simulink model "coffe"  (R2015a)
settings: Solver=ode45  StartTime=0.0  StopTime=10.0  RelTol=1e-3
settings Model: Creator=lenovo  LastModifiedBy=lenovo

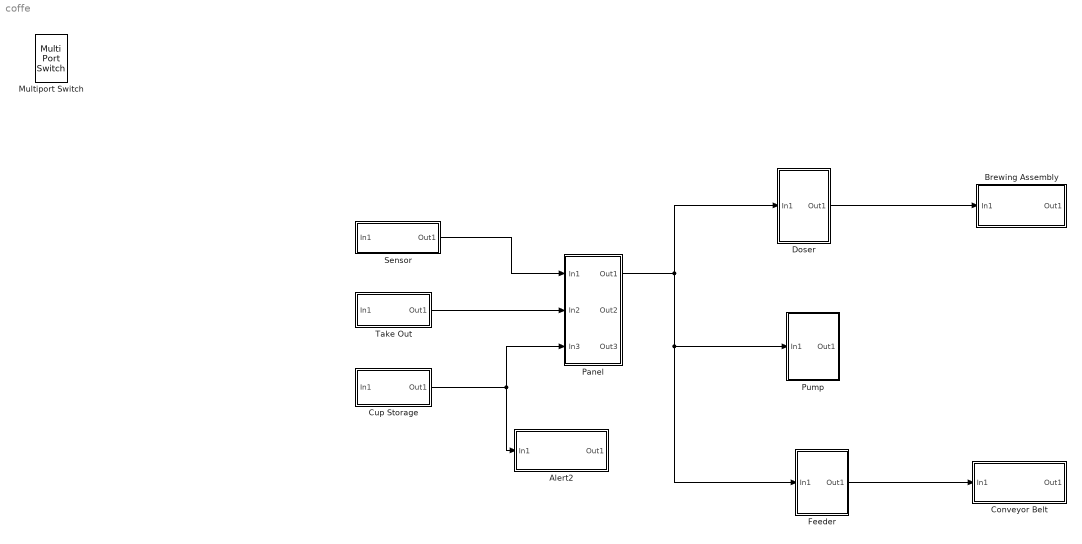
== system coffe ==
  Alert2 : Subsystem
  Brewing Assembly : Subsystem
  "Conveyor Belt " : Subsystem
  Cup Storage : Subsystem
  Doser : Subsystem
  Feeder : Subsystem
  Multiport Switch : MultiPortSwitch
  Panel : Subsystem
  Pump : Subsystem
  Sensor : Subsystem
  Take Out : Subsystem
  wires:
  Panel/1(Out1) -> Doser/1(In1), Feeder/1(In1), Pump/1(In1)
  Take Out/1(Out1) -> Panel/2(In2)
  Cup Storage/1(Out1) -> Panel/3(In3), Alert2/1(In1)
  Feeder/1(Out1) -> "Conveyor Belt "/1(In1)
  Doser/1(Out1) -> Brewing Assembly/1(In1)
  Sensor/1(Out1) -> Panel/1(In1)

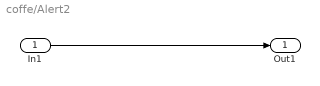
== system coffe/Alert2 ==
  In1 : Inport
  Out1 : Outport
  wires:
  In1/1 -> Out1/1

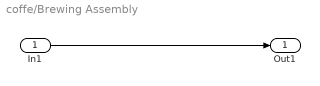
== system coffe/Brewing Assembly ==
  In1 : Inport
  Out1 : Outport
  wires:
  In1/1 -> Out1/1

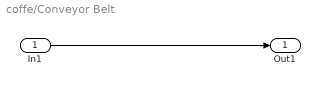
== system coffe/Conveyor Belt  ==
  In1 : Inport
  Out1 : Outport
  wires:
  In1/1 -> Out1/1

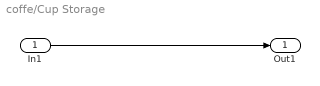
== system coffe/Cup Storage ==
  In1 : Inport
  Out1 : Outport
  wires:
  In1/1 -> Out1/1

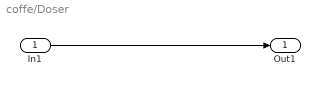
== system coffe/Doser ==
  In1 : Inport
  Out1 : Outport
  wires:
  In1/1 -> Out1/1

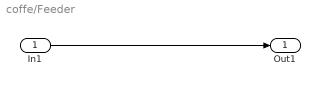
== system coffe/Feeder ==
  In1 : Inport
  Out1 : Outport
  wires:
  In1/1 -> Out1/1

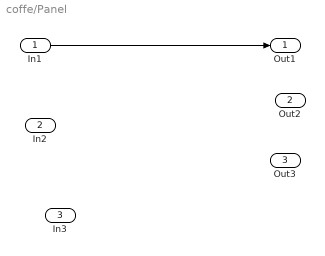
== system coffe/Panel ==
  In1 : Inport
  In2 : Inport  Port=2
  In3 : Inport  Port=3
  Out1 : Outport
  Out2 : Outport  Port=2
  Out3 : Outport  Port=3
  wires:
  In1/1 -> Out1/1

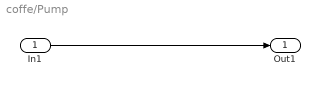
== system coffe/Pump ==
  In1 : Inport
  Out1 : Outport
  wires:
  In1/1 -> Out1/1

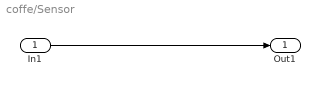
== system coffe/Sensor ==
  In1 : Inport
  Out1 : Outport
  wires:
  In1/1 -> Out1/1

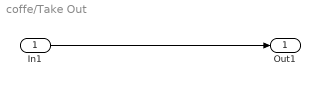
== system coffe/Take Out ==
  In1 : Inport
  Out1 : Outport
  wires:
  In1/1 -> Out1/1
